simulink model "PlantaOficial"  (R2024b)
settings: Solver=ode23tb  StartTime=0.0  StopTime=39  RelTol=1e-3
values from neighbouring files (symbols this model uses):
  C1 = 1.2801    [CodigoSavePoint.m]    (also in CodigoVT.m)
  C2 = 23.99    [CodigoSavePoint.m]    (also in CodigoVT.m)
  C3 = 0.52    [CodigoSavePoint.m]    (also in CodigoVT.m)
  VelRef = 17    [CodigoSavePoint.m]    (also in CodigoVT.m = 30)
undefined symbols (not defined in the file or in its folder): EV, fractalcoef, MTR
libraries: autolibmappedmotor x2, vrlib x1, slpidlib x1, mspsensorlib x1, vehdynlibviscommon x1, vehdynlibtire x1, vehdynlibscenariocommon x1, vehdynlibsteering x1, vehdynlibdriver x1, autolibshared x1
(part 2 of 2)

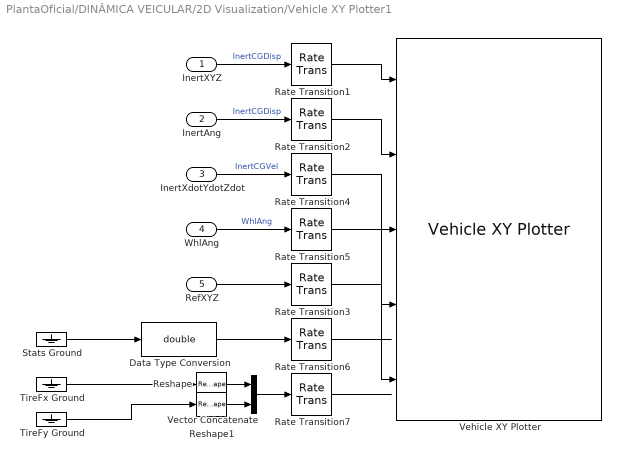
== system PlantaOficial/DINÂMICA VEICULAR/2D Visualization/Vehicle XY Plotter1 ==
  InertXYZ : Inport
  InertAng : Inport  Port=2
  InertXdotYdotZdot : Inport  Port=3
  WhlAng : Inport  Port=4
  RefXYZ : Inport  Port=5
  Data Type Conversion : DataTypeConversion  OutDataTypeStr=double  SaturateOnIntegerOverflow=off  RndMeth=Floor
  Rate Transition{1..7} (7 alike) : RateTransition  Deterministic=off  OutPortSampleTime=pltDT
  Reshape : Reshape  OutputDimensionality=Row vector (2-D)
  Reshape1 : Reshape  OutputDimensionality=Row vector (2-D)
  Stats Ground : Ground
  TireFx Ground : Ground
  TireFy Ground : Ground
  Vector Concatenate : Concatenate  Mode=Multidimensional array
  Vehicle XY Plotter : vehdynlibviscommon/Vehicle XY Plotter  w=w  a=a  b=b  figBorder=figBorder  bufferSize=bufferSize  extStats=off  extTireF=off
  wires:
  Vector Concatenate/1 -> Rate Transition7/1
  Reshape1/1 -> Vector Concatenate/2
  Reshape/1 -> Vector Concatenate/1
  RefXYZ/1 -> Rate Transition3/1
  Rate Transition7/1 -> ?
  Data Type Conversion/1 -> Rate Transition6/1
  Rate Transition6/1 -> ?
  Rate Transition5/1 -> Vehicle XY Plotter/4
  Rate Transition4/1 -> Vehicle XY Plotter/3
  Rate Transition2/1 -> Vehicle XY Plotter/2
  Rate Transition1/1 -> Vehicle XY Plotter/1
  Rate Transition3/1 -> Vehicle XY Plotter/5
  WhlAng/1 -> Rate Transition5/1  "WhlAng"
  InertXYZ/1 -> Rate Transition1/1  "InertCGDisp"
  InertXdotYdotZdot/1 -> Rate Transition4/1  "InertCGVel"
  InertAng/1 -> Rate Transition2/1  "InertCGDisp"
  Stats Ground/1 -> Data Type Conversion/1
  TireFx Ground/1 -> Reshape/1
  TireFy Ground/1 -> Reshape1/1
